simulink model "XSWIFT_cruise"  (R2025b)
settings: Solver=ode4  StartTime=0.0  StopTime=85  FixedStep=0.001  MaxStep=0.001  RelTol=1e-4
InitFcn:
  | [filepath, name] = fileparts(get_param(bdroot, 'FileName'))
  | if strcmp(filepath, pwd) ~= 1
  |     disp(strcat('cambiando el directorio actual a ', filepath))
  |     cd(filepath);
  | end
  | run(strcat(name, '_init'));
  | load("long_cruise.mat");
  | load("lat_cruise.mat")
values from neighbouring files (symbols this model uses):
  d2r = pi/180    (= 0.0174532925199)    [XSWIFT_cruise_init.m]
  data =     [XSWIFT_data.mat]
  init =     [XSWIFT_nav.mat]
  masa = data.mass.zfw + (data.mass.max_takeoff - data.mass.zfw) * mass_frac    [XSWIFT_cruise_init.m]
  nav =     [XSWIFT_nav.mat]
  obs_alpha_la = 20    [implementacion_digital_controles.m]    (also in long_cruise.mat)
  r = rad2deg(x(:,3))    [latero_direccional_LQR.m]
  r2d = 180/pi    (= 57.2957795131)    [XSWIFT_cruise_init.m]
  T_rec = 1/20    (= 0.05)    [XSWIFT_cruise_init.m]
  tau_filtro_lat = 0.3    [lat_cruise.mat]    (also in latero_direccional_LQR.m)
  Tc = 1/25    (= 0.04)    [XSWIFT_cruise_init.m]
  timeSince1970 = 1.3201e+09    (= 1320100000)    [XSWIFT_cruise_init.m]
  x_cg = 0    [XSWIFT_cruise_init.m]
  x_ref = 0    [XSWIFT_cruise_init.m]
undefined symbols (not defined in the file or in its folder): Earth, engine, F, m, MIL, Moderate, s, WGS84, wind
libraries: simulink x6, aerolibconvert2 x4, aerolibasang x4, aerolibfltsims x4, aerolibactuator x3, aerolibwind2 x2, aerolib6dof2 x1, aerolibadyn x1, aerolibatmos2 x1, aerolibanimutils x1, aerolibconvert x1, aerolibobsolete x1
(part 1 of 2)
settings Model: Creator=augusto  LastModifiedBy=Allan
settings SolverCC: AlgebraicLoopSolver=TrustRegion
settings DataIOCC: ReturnWorkspaceOutputs=off
settings DebuggingCC: UnconnectedInputMsg=warning  UnconnectedOutputMsg=warning  UnconnectedLineMsg=warning  ArithmeticOperatorsInVariantConditions=warning
settings ModelReferenceCC: EnableRefExpFcnMdlSchedulingChecks=on
settings SFSimCC: SimUseLocalCustomCode=off  CustomCodeUndefinedFunction=UseInterfaceOnly
settings RTWCC: RTWUseLocalCustomCode=off  GPUComputeCapability=3.5
settings CodeAppCC: StateflowObjectComments=on

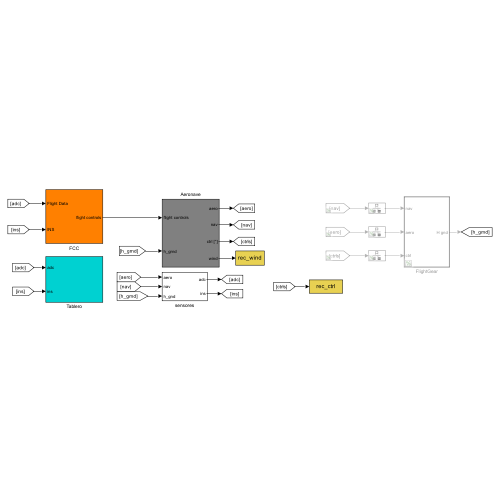
[thumbnail: Simulink's stored preview of the top-level diagram]
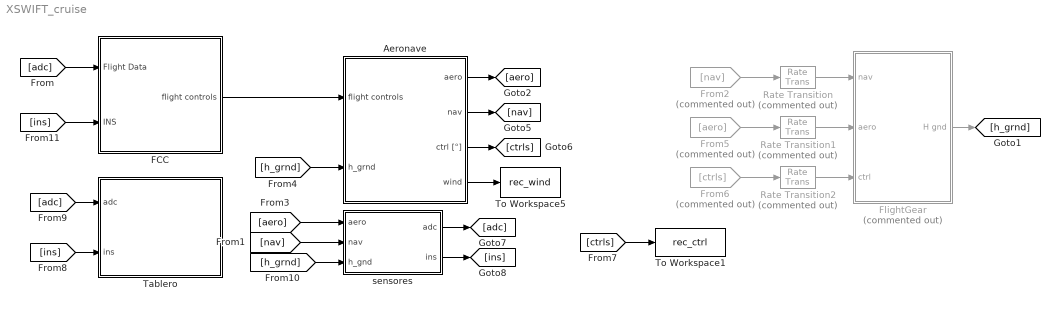
== system XSWIFT_cruise ==
  Aeronave : Subsystem
  FCC : Subsystem
  FlightGear : Subsystem  Commented=on  TreatAsAtomicUnit=on  VariantControl=FlightGearVariant
  From2 : From  Commented=on  GotoTag=nav
  From5 : From  Commented=on  GotoTag=aero
  From6 : From  Commented=on  GotoTag=ctrls
  Rate Transition : RateTransition  Commented=on
  Rate Transition1 : RateTransition  Commented=on
  Rate Transition2 : RateTransition  Commented=on
  Tablero : Subsystem
  To Workspace1 : ToWorkspace  VariableName=rec_ctrl  SampleTime=T_rec
      settings: MaxDataPoints=N_rec
  To Workspace5 : ToWorkspace  VariableName=rec_wind  SampleTime=T_rec
      settings: MaxDataPoints=N_rec
  sensores : Subsystem
  wires:
  FlightGear/1(H gnd) -> [h_grnd]
  From5/1 -> Rate Transition1/1
  Rate Transition2/1 -> FlightGear/3(ctrl)
  Rate Transition1/1 -> FlightGear/2(aero)
  From2/1 -> Rate Transition/1
  From6/1 -> Rate Transition2/1
  Rate Transition/1 -> FlightGear/1(nav)
  [adc] -> FCC/1(Flight Data)
  [ins] -> FCC/2(INS)
  [adc] -> Tablero/1(adc)
  [ins] -> Tablero/2(ins)
  [h_grnd] -> Aeronave/2(h_grnd)
  FCC/1(flight controls) -> Aeronave/1(flight controls)
  Aeronave/3(ctrl [°]) -> [ctrls]
  Aeronave/4(wind) -> To Workspace5/1
  sensores/1(adc) -> [adc]
  sensores/2(ins) -> [ins]
  Aeronave/1(aero) -> [aero]
  Aeronave/2(nav) -> [nav]
  [aero] -> sensores/1(aero)
  [nav] -> sensores/2(nav)
  [h_grnd] -> sensores/3(h_gnd)
  [ctrls] -> To Workspace1/1

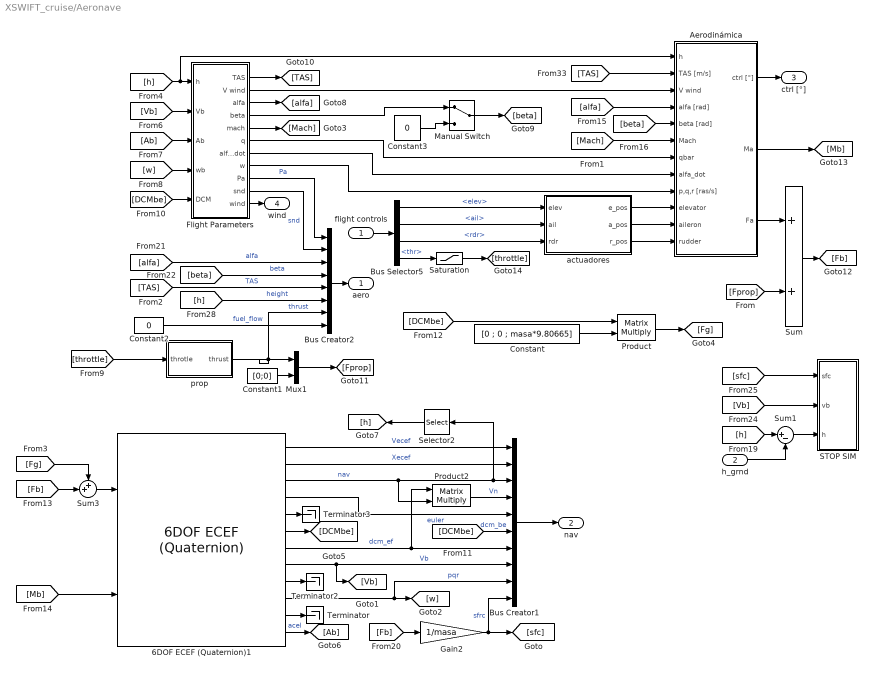
== system XSWIFT_cruise/Aeronave ==
  flight controls : Inport
  h_grnd : Inport  Port=2
  6DOF ECEF (Quaternion)1 : aerolib6dof2/6DOF ECEF (Quaternion)  units=Metric (MKS)  mtype=Fixed  xg_0=init.lla  Vm_0=init.vb  eul_0=init.eul  pm_0=init.wb  mass_0=masa  mass_e=0.5  mass_f=2.0  inertia=inercia  inertia_e=eye(3)  inertia_f=2*eye(3)  vre_flag=on  abi_flag=off  ptype=Earth (WGS84)  R=6378137  F=1/298.257223563  w_E=7292115e-11  angle_in=Internal  LPM0=0  quat_statename=''  pm_statename=''  Vm_statename=''  posfixedframe_statename=''  posinertial_statename=''  LPM_statename=''  mass_statename=''
  Aerodinámica : Subsystem
  Bus Creator1 : BusCreator  Inputs=10
  Bus Creator2 : BusCreator  Inputs=8
  Bus Selector5 : BusSelector  OutputSignals=elev,ail,rdr,thr
  Constant : Constant  Value=[0 ; 0 ; masa*9.80665]
  Constant1 : Constant  Value=[0;0]
  Constant2 : Constant  Value=0
  Constant3 : Constant  Value=0
  Flight Parameters : Subsystem
  Gain2 : Gain  Gain=1/masa
  Manual Switch : ManualSwitch
  Mux1 : Mux  Inputs=2
  Product : Product  Multiplication=Matrix(*)  RndMeth=Zero
  Product2 : Product  Multiplication=Matrix(*)  RndMeth=Zero
  STOP SIM : Subsystem
  Saturation : Saturate  UpperLimit=1  LowerLimit=0
  Selector2 : Selector  InputPortWidth=3  IndexOptions=Index vector (dialog)  Indices=[3]  OutputSizes=1
  Sum : Sum
  Sum1 : Sum  Inputs=|+-
  Sum3 : Sum  Inputs=++|
  Terminator : Terminator
  Terminator2 : Terminator
  Terminator3 : Terminator
  actuadores : Subsystem
  prop : Subsystem
  aero : Outport
  nav : Outport  Port=2
  ctrl [°] : Outport  Port=3
  wind : Outport  Port=4
  wires:
  6DOF ECEF (Quaternion)1/2 -> Bus Creator1/2  "Xecef"
  6DOF ECEF (Quaternion)1/6 -> [DCMbe]
  6DOF ECEF (Quaternion)1/8 -> [Vb], Bus Creator1/8  "Vb"
  6DOF ECEF (Quaternion)1/9 -> Terminator2/1
  6DOF ECEF (Quaternion)1/12 -> [Ab]  "acel"
  Constant/1 -> Product/2
  Constant2/1 -> Bus Creator2/8  "fuel_flow"
  Constant1/1 -> Mux1/2
  [h] -> Aerodinámica/1(h), Flight Parameters/1(h)
  [Vb] -> Flight Parameters/2(Vb)
  Flight Parameters/6(q) -> Aerodinámica/7(qbar)
  Flight Parameters/5(mach) -> [Mach]
  [Mach] -> Aerodinámica/6(Mach)
  Flight Parameters/3(alfa) -> [alfa]
  [alfa] -> Aerodinámica/4(alfa [rad])
  [beta] -> Aerodinámica/5(beta [rad])
  Flight Parameters/2(V wind) -> Aerodinámica/3(V wind)
  Aerodinámica/3(Fa) -> Sum/1
  Flight Parameters/1(TAS) -> [TAS]
  6DOF ECEF (Quaternion)1/4 -> Bus Creator1/5  "euler"
  [Ab] -> Flight Parameters/3(Ab)
  Flight Parameters/7(alfa_dot) -> Aerodinámica/8(alfa_dot)
  Sum/1 -> [Fb]
  6DOF ECEF (Quaternion)1/10 -> Bus Creator1/9, [w]  "pqr"
  [alfa] -> Bus Creator2/3  "alfa"
  [beta] -> Bus Creator2/4  "beta"
  [TAS] -> Bus Creator2/5  "TAS"
  Bus Creator2/1 -> aero/1
  Bus Selector5/4 -> Saturation/1  "<thr>"
  Flight Parameters/8(w) -> Aerodinámica/9(p,q,r [ras/s])
  [w] -> Flight Parameters/4(wb)
  [DCMbe] -> Flight Parameters/5(DCM)
  [DCMbe] -> Bus Creator1/6  "dcm_be"
  Saturation/1 -> [throttle]
  Aerodinámica/2(Ma) -> [Mb]
  6DOF ECEF (Quaternion)1/5 -> Terminator3/1
  6DOF ECEF (Quaternion)1/3 -> Product2/2, Bus Creator1/3, Selector2/1  "nav"
  Aerodinámica/1(ctrl [°]) -> ctrl [°]/1
  Bus Creator1/1 -> nav/1
  Flight Parameters/9(Pa) -> Bus Creator2/1  "Pa"
  6DOF ECEF (Quaternion)1/7 -> Bus Creator1/7, Product2/1  "dcm_ef"
  Product2/1 -> Bus Creator1/4  "Vn"
  6DOF ECEF (Quaternion)1/1 -> Bus Creator1/1  "Vecef"
  flight controls/1 -> Bus Selector5/1
  [h] -> Bus Creator2/6  "height"
  Flight Parameters/10(snd) -> Bus Creator2/2  "snd"
  [Fb] -> Gain2/1
  Gain2/1 -> [sfc], Bus Creator1/10  "sfrc"
  Flight Parameters/11(wind) -> wind/1
  Selector2/1 -> [h]
  [TAS] -> Aerodinámica/2(TAS [m/s])
  Bus Selector5/1 -> actuadores/1(elev)  "<elev>"
  Bus Selector5/2 -> actuadores/2(ail)  "<ail>"
  Bus Selector5/3 -> actuadores/3(rdr)  "<rdr>"
  actuadores/1(e_pos) -> Aerodinámica/10(elevator)
  actuadores/2(a_pos) -> Aerodinámica/11(aileron)
  actuadores/3(r_pos) -> Aerodinámica/12(rudder)
  Product/1 -> [Fg]
  [Fb] -> Sum3/2
  [Fg] -> Sum3/1
  [DCMbe] -> Product/1
  Sum3/1 -> 6DOF ECEF (Quaternion)1/1
  [throttle] -> prop/1(throtle)
  prop/1(thrust) -> Mux1/1, Bus Creator2/7  "thrust"
  [Mb] -> 6DOF ECEF (Quaternion)1/2
  [sfc] -> STOP SIM/1(sfc)
  [Vb] -> STOP SIM/2(vb)
  [Fprop] -> Sum/2
  Mux1/1 -> [Fprop]
  [h] -> Sum1/1
  Sum1/1 -> STOP SIM/3(h)
  h_grnd/1 -> Sum1/2
  6DOF ECEF (Quaternion)1/11 -> Terminator/1
  Manual Switch/1 -> [beta]
  Flight Parameters/4(beta) -> Manual Switch/1
  Constant3/1 -> Manual Switch/2

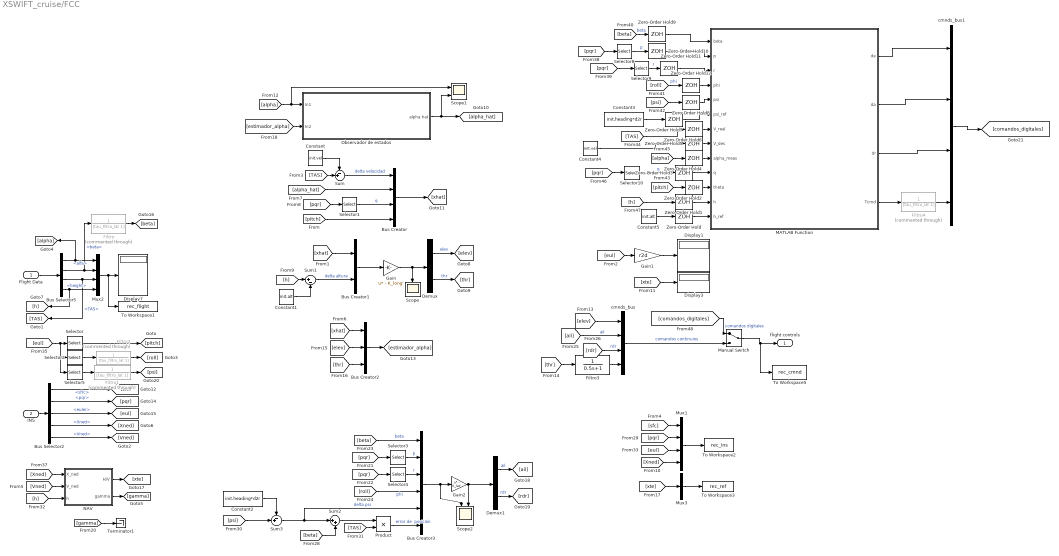
== system XSWIFT_cruise/FCC ==
  Flight Data : Inport
  INS : Inport  Port=2
  Bus Selector2 : BusSelector  OutputSignals=sfrc,pqr,euler,Xned,Vned
  Bus Selector5 : BusSelector  OutputSignals=alfa,beta,TAS,height
  Bus Creator : BusCreator  Inputs=4
  Bus Creator1 : BusCreator  Inputs=2
  Bus Creator2 : BusCreator  Inputs=3
  Bus Creator3 : BusCreator  Inputs=6
  Constant : Constant  Value=init.vel
  Constant1 : Constant  Value=init.alt
  Constant2 : Constant  Value=init.heading*d2r
  Constant3 : Constant  Value=init.heading*d2r
  Constant4 : Constant  Value=init.vel
  Constant5 : Constant  Value=init.alt
  Demux : Demux  Outputs=2
  Demux1 : Demux  Outputs=2
  Display1 : Display
  Display3 : Display
  Display7 : Display
  Filtro{,1..2,4} (4 alike) : TransferFcn  Commented=through  Denominator=[tau_filtro_lat 1]
  Filtro3 : TransferFcn  Denominator=[0.5 1]
  Gain : Gain  Gain=- K_long'  Multiplication=Matrix(u*K)
  Gain1 : Gain  Gain=r2d
  Gain2 : Gain  Gain=- K_lat'  Multiplication=Matrix(u*K)
  MATLAB Function : MATLAB Function  TreatAsAtomicUnit=on
  Manual Switch : ManualSwitch
  Mux1 : Mux
  Mux2 : Mux
  Mux3 : Mux  Inputs=1
  NAV : Subsystem
  Observador de estados : Subsystem
  Product : Product
  Scope : Scope
      settings: ActiveDisplayYMinimum=-0.63580956795157817  ActiveDisplayYMaximum=2.7800022979084402
  Scope1 : Scope  NumInputPorts=2
      settings: ActiveDisplayYMinimum=-0.053966559568766573  ActiveDisplayYMaximum=-0.02656502251691319  DataLoggingVariableName=ScopeData2
  Scope2 : Scope  NumInputPorts=2
      settings: ActiveDisplayYMinimum=-6.3589608284384154  ActiveDisplayYMaximum=1.5540132529438384  DataLoggingVariableName=ScopeData3
  Selector : Selector  InputPortWidth=3  IndexOptions=Index vector (dialog)  Indices=2  OutputSizes=1
  Selector1 : Selector  InputPortWidth=3  IndexOptions=Index vector (dialog)  Indices=2  OutputSizes=1
  Selector10 : Selector  InputPortWidth=3  IndexOptions=Index vector (dialog)  Indices=2  OutputSizes=1
  Selector2 : Selector  InputPortWidth=3  IndexOptions=Index vector (dialog)  Indices=1  OutputSizes=1
  Selector3 : Selector  InputPortWidth=3  IndexOptions=Index vector (dialog)  Indices=1  OutputSizes=1
  Selector4 : Selector  InputPortWidth=3  IndexOptions=Index vector (dialog)  Indices=3  OutputSizes=1
  Selector5 : Selector  InputPortWidth=3  IndexOptions=Index vector (dialog)  Indices=3  OutputSizes=1
  Selector8 : Selector  InputPortWidth=3  IndexOptions=Index vector (dialog)  Indices=1  OutputSizes=1
  Selector9 : Selector  InputPortWidth=3  IndexOptions=Index vector (dialog)  Indices=3  OutputSizes=1
  Sum : Sum  Inputs=-+|
  Sum1 : Sum  Inputs=|+-
  Sum2 : Sum  Inputs=|++
  Sum3 : Sum  Inputs=-+|
  Terminator1 : Terminator
  To Workspace1 : ToWorkspace  VariableName=rec_flight  SampleTime=T_rec
      settings: MaxDataPoints=N_rec
  To Workspace2 : ToWorkspace  VariableName=rec_ins  SampleTime=T_rec
      settings: MaxDataPoints=N_rec
  To Workspace3 : ToWorkspace  VariableName=rec_ref  SampleTime=T_rec
      settings: MaxDataPoints=N_rec
  To Workspace5 : ToWorkspace  VariableName=rec_cmnd  SampleTime=T_rec
      settings: MaxDataPoints=N_rec
  Zero-Order Hold{,1..12} (13 alike) : ZeroOrderHold  SampleTime=-1
  cmnds_bus : BusCreator  Inputs=4  OutDataTypeStr=Bus: cmnds_bus
      settings: InheritFromInputs=off
  cmnds_bus1 : BusCreator  Inputs=4  OutDataTypeStr=Bus: cmnds_bus
      settings: InheritFromInputs=off
  flight controls : Outport
  wires:
  Mux2/1 -> To Workspace1/1, Display7/1
  Bus Selector5/2 -> Filtro/1, Mux2/2  "<beta>"
  Bus Selector5/1 -> [alpha], Mux2/1  "<alfa>"
  Bus Selector5/3 -> [TAS], Mux2/3  "<TAS>"
  Bus Selector5/4 -> [h], Mux2/4  "<height>"
  INS/1 -> Bus Selector2/1
  Flight Data/1 -> Bus Selector5/1
  [rdr] -> cmnds_bus/3  "rdr"
  [ail] -> cmnds_bus/2  "ail"
  Bus Selector2/3 -> [eul]  "<euler>"
  Selector/1 -> [pitch]
  Bus Selector2/1 -> [sfc]  "<sfrc>"
  Bus Selector2/2 -> [pqr]  "<pqr>"
  [Xned] -> Mux1/4
  [xte] -> Display3/1
  Mux3/1 -> To Workspace3/1
  [xte] -> Mux3/1
  Bus Selector2/4 -> [Xned]  "<Xned>"
  Mux1/1 -> To Workspace2/1
  [sfc] -> Mux1/1
  [pqr] -> Mux1/2
  [eul] -> Mux1/3
  Gain1/1 -> Display1/1
  [eul] -> Gain1/1
  [pitch] -> Bus Creator/4
  [Xned] -> NAV/1(X_ned)
  NAV/1(H/V) -> [xte]
  [h] -> NAV/3(h)
  Bus Selector2/5 -> [Vned]  "<Vned>"
  [Vned] -> NAV/2(V_ned)
  NAV/2(gamma) -> [gamma]
  [alpha_hat] -> Bus Creator/2
  [pqr] -> Selector1/1
  Selector1/1 -> Bus Creator/3  "q"
  Bus Creator1/1 -> Gain/1
  [h] -> Sum1/1
  Gain/1 -> Scope/1, Demux/1
  Demux/1 -> [elev]  "elev"
  Demux/2 -> [thr]  "thr"
  [TAS] -> Sum/2
  Sum/1 -> Bus Creator/1  "delta velocidad"
  Sum1/1 -> Bus Creator1/2  "delta altura"
  Constant1/1 -> Sum1/2
  [elev] -> cmnds_bus/1
  [thr] -> Filtro3/1
  Bus Creator/1 -> [xhat]
  [xhat] -> Bus Creator1/1
  [xhat] -> Bus Creator2/1
  [elev] -> Bus Creator2/2
  [thr] -> Bus Creator2/3
  Bus Creator2/1 -> [estimador_alpha]
  [alpha] -> Scope1/1, Observador de estados/1(In1)
  Observador de estados/1(alpha hat) -> [alpha_hat], Scope1/2
  [estimador_alpha] -> Observador de estados/2(In2)
  [gamma] -> Terminator1/1
  Constant/1 -> Sum/1
  [pqr] -> Selector3/1
  [pqr] -> Selector4/1
  [beta] -> Bus Creator3/1  "beta"
  Selector3/1 -> Bus Creator3/2  "p"
  Selector4/1 -> Bus Creator3/3  "r"
  [roll] -> Bus Creator3/4  "phi"
  Demux1/2 -> [rdr]  "rdr"
  Gain2/1 -> Demux1/1, Scope2/2
  Demux1/1 -> [ail]  "ail"
  Bus Creator3/1 -> Scope2/1, Gain2/1
  [eul] -> Selector5/1, Selector2/1, Selector/1
  [beta] -> Sum2/2
  Sum2/1 -> Product/1
  [TAS] -> Product/2
  [psi] -> Sum3/2
  Constant2/1 -> Sum3/1
  Sum3/1 -> Sum2/1, Bus Creator3/5  "delta psi"
  Product/1 -> Bus Creator3/6  "error de  posición"
  Filtro/1 -> [beta]
  Selector5/1 -> Filtro1/1
  Filtro1/1 -> [psi]
  Selector2/1 -> Filtro2/1
  Filtro2/1 -> [roll]
  [pqr] -> Selector8/1
  [roll] -> Zero-Order Hold12/1  "phi"
  Selector9/1 -> Zero-Order Hold11/1  "r"
  [beta] -> Zero-Order Hold9/1  "beta"
  Selector8/1 -> Zero-Order Hold10/1  "p"
  [pqr] -> Selector9/1
  [psi] -> Zero-Order Hold8/1
  Constant3/1 -> Zero-Order Hold7/1
  Constant4/1 -> Zero-Order Hold5/1
  [pqr] -> Selector10/1
  [TAS] -> Zero-Order Hold6/1
  [pitch] -> Zero-Order Hold2/1
  Selector10/1 -> Zero-Order Hold3/1  "q"
  [alpha] -> Zero-Order Hold4/1
  [h] -> Zero-Order Hold1/1
  Constant5/1 -> Zero-Order Hold/1
  MATLAB Function/4(Tcmd) -> Filtro4/1
  cmnds_bus1/1 -> [comandos_digitales]
  [comandos_digitales] -> Manual Switch/1  "comandos digitales"
  Zero-Order Hold/1 -> MATLAB Function/13(h_ref)
  Zero-Order Hold1/1 -> MATLAB Function/12(h)
  Zero-Order Hold2/1 -> MATLAB Function/11(theta)
  Zero-Order Hold3/1 -> MATLAB Function/10(q)
  Zero-Order Hold4/1 -> MATLAB Function/9(alpha_meas)
  Zero-Order Hold5/1 -> MATLAB Function/8(V_des)
  Zero-Order Hold6/1 -> MATLAB Function/7(V_real)
  Zero-Order Hold7/1 -> MATLAB Function/6(psi_ref)
  Zero-Order Hold8/1 -> MATLAB Function/5(psi)
  Zero-Order Hold9/1 -> MATLAB Function/1(beta)
  Zero-Order Hold10/1 -> MATLAB Function/2(p)
  Zero-Order Hold11/1 -> MATLAB Function/3(r)
  Zero-Order Hold12/1 -> MATLAB Function/4(phi)
  MATLAB Function/1(de) -> cmnds_bus1/1
  MATLAB Function/2(da) -> cmnds_bus1/2
  MATLAB Function/3(dr) -> cmnds_bus1/3
  cmnds_bus/1 -> Manual Switch/2  "comandos continuios"
  Manual Switch/1 -> To Workspace5/1, flight controls/1
  Filtro3/1 -> cmnds_bus/4
  Filtro4/1 -> cmnds_bus1/4

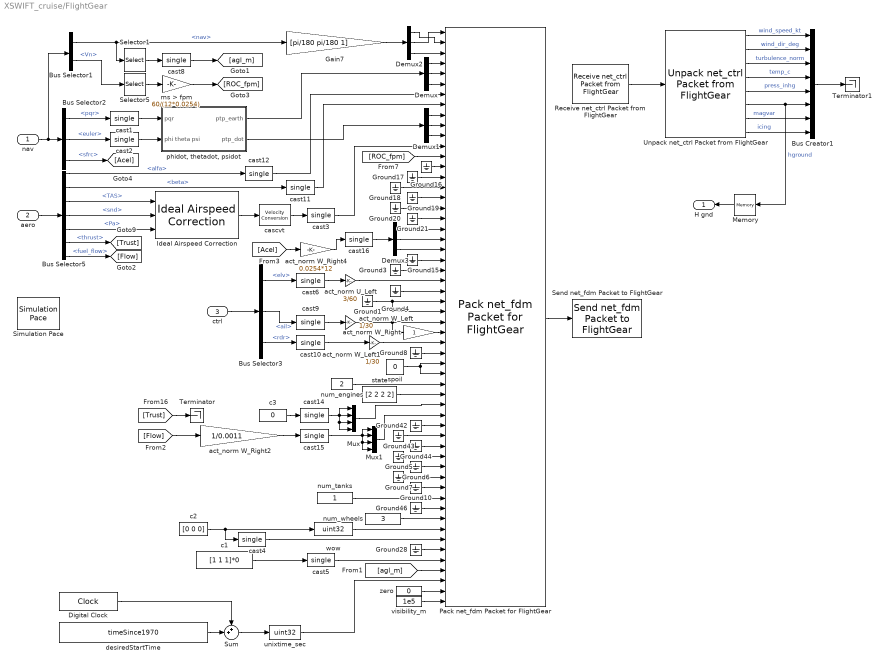
== system XSWIFT_cruise/FlightGear ==
  nav : Inport  SampleTime=Tc
  aero : Inport  Port=2  SampleTime=Tc
  ctrl : Inport  Port=3  SampleTime=Tc
  Bus Creator1 : BusCreator  Inputs=8
  Bus Selector1 : BusSelector  OutputSignals=nav,Vn
  Bus Selector2 : BusSelector  OutputSignals=pqr,euler,sfrc
  Bus Selector3 : BusSelector  OutputSignals=elv,ail,rdr
  Bus Selector5 : BusSelector  OutputSignals=alfa,beta,TAS,snd,Pa,thrust,fuel_flow
  Demux{,1..3} (4 alike) : Demux  Outputs=3
  Digital Clock : DigitalClock  SampleTime=Tc
  Gain7 : Gain  Gain=[pi/180 pi/180 1]
  Ground{1,3..8,10,15..21,28,42..44,46} (20 alike) : Ground
  Ideal Airspeed Correction : aerolibasang/Ideal Airspeed Correction  units=Metric (MKS)  vel_in=TAS  vel_out_tas=CAS  vel_out_eas=CAS  vel_out_cas=TAS  method=Table Lookup  SubOnly=off  action=Warning
  Memory : Memory  InheritSampleTime=on
  Mux : Mux
  Mux1 : Mux
  Pack net_fdm Packet for FlightGear : aerolibfltsims/Pack net_fdm Packet for FlightGear  FlightGearVersion=v2016.3  ShowPositionAttitudeInputs=on  ShowVelocityAccelerationInputs=on  ShowControlSurfacePositionInputs=on  ShowEngineFuelInputs=on  ShowLandingGearInputs=on  ShowEnvironmentInputs=on  SampleTime=Tc  packetVersion=24
  Receive net_ctrl Packet from FlightGear : aerolibfltsims/Receive net_ctrl Packet from FlightGear  FlightGearVersion=v3.0  ReceiveAddress=127.0.0.1  ReceivePort=5505  ReceiveWidth=744  varLen=off  SampleTime=Tc  packetFlag=off
      settings: AttributesFormatString=Version Selected:\n%<FlightGearVersion>
  Selector1 : Selector  InputPortWidth=3  IndexOptions=Index vector (dialog)  Indices=3  OutputSizes=1
  Selector5 : Selector  InputPortWidth=3  IndexOptions=Index vector (dialog)  Indices=3  OutputSizes=1
  Send net_fdm Packet to FlightGear : aerolibfltsims/Send net_fdm Packet to FlightGear  DestinationIpAddress=127.0.0.1  DestinationPort=5502  LocalIpPort=-1  varLen=off  SampleTime=Tc
  Simulation Pace : aerolibanimutils/Simulation Pace  SimulationPace=1  SleepMode=MATLAB Thread  OutputPaceError=off  SampleTime=Tc
      settings: AttributesFormatString=%<SimulationPace> sec/sec
  Sum : Sum  Inputs=++|
  Terminator : Terminator
  Terminator1 : Terminator
  Unpack net_ctrl Packet from FlightGear : aerolibfltsims/Unpack net_ctrl Packet from FlightGear  FlightGearVersion=v2016.3  ShowControlSurfacePositionOutputs=off  ShowEngineFuelOutputs=off  ShowLandingGearOutputs=off  ShowAvionicOutputs=off  ShowEnvironmentOutputs=on  SampleTime=Tc  packetVersion=27
      settings: AttributesFormatString=Version Selected: %<FlightGearVersion>
  act_norm U_Left : Gain  Gain=3/60
      settings: AttributesFormatString=%<Gain>
  act_norm W_Left : Gain  Gain=1/30
      settings: AttributesFormatString=%<Gain>
  act_norm W_Left1 : Gain  Gain=1/30
      settings: AttributesFormatString=%<Gain>
  act_norm W_Right : Gain
      settings: AttributesFormatString=%<Gain>
  act_norm W_Right2 : Gain  Gain=1/0.0011
      settings: AttributesFormatString=%<Gain>
  act_norm W_Right4 : Gain  Gain=0.0254*12
      settings: AttributesFormatString=%<Gain>
  c1 : Constant  Value=[1 1 1]*0  OutDataTypeStr=uint32
  c2 : Constant  Value=[0 0 0]  OutDataTypeStr=uint32
  c3 : Constant  Value=0  OutDataTypeStr=uint32
  cascvt : aerolibconvert/Velocity Conversion  IU=m/s  OU=kts
  cast{1..6,8..12,14..16} (14 alike) : DataTypeConversion  OutDataTypeStr=single  RndMeth=Floor
  desiredStartTime : Constant  Value=timeSince1970
  ms > fpm : Gain  Gain=60/(12*0.0254)  OutDataTypeStr=single
  num_engines : Constant  Value=2  OutDataTypeStr=uint32
  num_tanks : Constant  OutDataTypeStr=uint32
  num_wheels : Constant  Value=3  OutDataTypeStr=uint32
  "phidot, thetadot, psidot" : Subsystem
  spoil : Constant  Value=0  OutDataTypeStr=single
  state : Constant  Value=[2 2 2 2]  OutDataTypeStr=uint32
  unixtime_sec : DataTypeConversion  OutDataTypeStr=uint32  RndMeth=Floor
  visibility_m : Constant  Value=1e5  OutDataTypeStr=single
  wow : DataTypeConversion  OutDataTypeStr=uint32  RndMeth=Floor
  zero : Constant  Value=0  OutDataTypeStr=int32
  H gnd : Outport
  wires:
  Unpack net_ctrl Packet from FlightGear/6 -> Memory/1, Bus Creator1/6  "hground"
  Unpack net_ctrl Packet from FlightGear/8 -> Bus Creator1/8  "icing"
  Unpack net_ctrl Packet from FlightGear/7 -> Bus Creator1/7  "magvar"
  Unpack net_ctrl Packet from FlightGear/5 -> Bus Creator1/5  "press_inhg"
  Unpack net_ctrl Packet from FlightGear/4 -> Bus Creator1/4  "temp_c"
  Unpack net_ctrl Packet from FlightGear/3 -> Bus Creator1/3  "turbulence_norm"
  Unpack net_ctrl Packet from FlightGear/2 -> Bus Creator1/2  "wind_dir_deg"
  Unpack net_ctrl Packet from FlightGear/1 -> Bus Creator1/1  "wind_speed_kt"
  Receive net_ctrl Packet from FlightGear/1 -> Unpack net_ctrl Packet from FlightGear/1
  Ground1/1 -> Pack net_fdm Packet for FlightGear/28, Pack net_fdm Packet for FlightGear/27
  Ground10/1 -> Pack net_fdm Packet for FlightGear/45
  wow/1 -> Pack net_fdm Packet for FlightGear/49
  cast9/1 -> act_norm W_Left/1
  Ground8/1 -> Pack net_fdm Packet for FlightGear/32
  act_norm W_Right/1 -> Pack net_fdm Packet for FlightGear/30
  act_norm W_Left/1 -> act_norm W_Right/1, Pack net_fdm Packet for FlightGear/29
  Ground4/1 -> Pack net_fdm Packet for FlightGear/26
  Ground7/1 -> Pack net_fdm Packet for FlightGear/44
  Ground6/1 -> Pack net_fdm Packet for FlightGear/43
  Ground5/1 -> Pack net_fdm Packet for FlightGear/42
  Ground3/1 -> Pack net_fdm Packet for FlightGear/24
  Demux1/3 -> Pack net_fdm Packet for FlightGear/11
  Demux1/2 -> Pack net_fdm Packet for FlightGear/10
  Demux1/1 -> Pack net_fdm Packet for FlightGear/9
  act_norm U_Left/1 -> Pack net_fdm Packet for FlightGear/25
  [agl_m] -> Pack net_fdm Packet for FlightGear/53
  Demux/3 -> Pack net_fdm Packet for FlightGear/6
  Demux/2 -> Pack net_fdm Packet for FlightGear/5
  Demux/1 -> Pack net_fdm Packet for FlightGear/4
  cast4/1 -> Pack net_fdm Packet for FlightGear/50
  cast6/1 -> act_norm U_Left/1
  cast5/1 -> Pack net_fdm Packet for FlightGear/52
  ms > fpm/1 -> [ROC_fpm]
  [ROC_fpm] -> Pack net_fdm Packet for FlightGear/13
  Bus Selector5/5 -> Ideal Airspeed Correction/3  "<Pa>"
  Bus Selector5/4 -> Ideal Airspeed Correction/2  "<snd>"
  Bus Selector2/2 -> cast2/1  "<euler>"
  Bus Selector2/1 -> cast1/1  "<pqr>"
  "phidot, thetadot, psidot"/2(ptp_dot) -> Demux1/1
  "phidot, thetadot, psidot"/1(ptp_earth) -> Demux/1
  cast3/1 -> Pack net_fdm Packet for FlightGear/12
  cast1/1 -> "phidot, thetadot, psidot"/1(pqr)
  cast2/1 -> "phidot, thetadot, psidot"/2(phi theta psi)
  visibility_m/1 -> Pack net_fdm Packet for FlightGear/56
  zero/1 -> Pack net_fdm Packet for FlightGear/55
  unixtime_sec/1 -> Pack net_fdm Packet for FlightGear/54
  Sum/1 -> unixtime_sec/1
  desiredStartTime/1 -> Sum/2
  Digital Clock/1 -> Sum/1
  cascvt/1 -> cast3/1
  Ideal Airspeed Correction/1 -> cascvt/1
  Ground28/1 -> Pack net_fdm Packet for FlightGear/51
  num_wheels/1 -> Pack net_fdm Packet for FlightGear/48
  Ground46/1 -> Pack net_fdm Packet for FlightGear/47
  num_tanks/1 -> Pack net_fdm Packet for FlightGear/46
  Ground44/1 -> Pack net_fdm Packet for FlightGear/41
  Ground43/1 -> Pack net_fdm Packet for FlightGear/40
  Ground42/1 -> Pack net_fdm Packet for FlightGear/39
  state/1 -> Pack net_fdm Packet for FlightGear/36
  num_engines/1 -> Pack net_fdm Packet for FlightGear/35
  Ground15/1 -> Pack net_fdm Packet for FlightGear/23
  Demux3/3 -> Pack net_fdm Packet for FlightGear/22
  Demux3/2 -> Pack net_fdm Packet for FlightGear/21
  Demux3/1 -> Pack net_fdm Packet for FlightGear/20
  Ground21/1 -> Pack net_fdm Packet for FlightGear/19
  Ground20/1 -> Pack net_fdm Packet for FlightGear/18
  Ground19/1 -> Pack net_fdm Packet for FlightGear/17
  Ground18/1 -> Pack net_fdm Packet for FlightGear/16
  Ground17/1 -> Pack net_fdm Packet for FlightGear/15
  Ground16/1 -> Pack net_fdm Packet for FlightGear/14
  Bus Selector3/1 -> cast6/1  "<elv>"
  Bus Selector3/2 -> cast9/1  "<ail>"
  cast10/1 -> act_norm W_Left1/1
  Bus Selector3/3 -> cast10/1  "<rdr>"
  act_norm W_Left1/1 -> Pack net_fdm Packet for FlightGear/31
  Demux2/3 -> Pack net_fdm Packet for FlightGear/3
  Bus Selector1/1 -> Gain7/1, Selector1/1  "<nav>"
  Bus Selector5/3 -> Ideal Airspeed Correction/1  "<TAS>"
  Selector5/1 -> ms > fpm/1
  Bus Selector1/2 -> Selector5/1  "<Vn>"
  c2/1 -> cast4/1, wow/1
  Selector1/1 -> cast8/1
  cast8/1 -> [agl_m]
  Gain7/1 -> Demux2/1
  Pack net_fdm Packet for FlightGear/1 -> Send net_fdm Packet to FlightGear/1
  Demux2/2 -> Pack net_fdm Packet for FlightGear/1
  Demux2/1 -> Pack net_fdm Packet for FlightGear/2
  Bus Selector5/2 -> cast11/1  "<beta>"
  cast12/1 -> Pack net_fdm Packet for FlightGear/7
  cast11/1 -> Pack net_fdm Packet for FlightGear/8
  Bus Selector5/1 -> cast12/1  "<alfa>"
  spoil/1 -> Pack net_fdm Packet for FlightGear/34, Pack net_fdm Packet for FlightGear/33
  Memory/1 -> H gnd/1
  Bus Creator1/1 -> Terminator1/1
  nav/1 -> Bus Selector2/1, Bus Selector1/1
  aero/1 -> Bus Selector5/1
  ctrl/1 -> Bus Selector3/1
  Bus Selector5/6 -> [Trust]  "<thrust>"
  Bus Selector5/7 -> [Flow]  "<fuel_flow>"
  act_norm W_Right2/1 -> cast15/1
  [Flow] -> act_norm W_Right2/1
  Bus Selector2/3 -> [Acel]  "<sfrc>"
  cast16/1 -> Demux3/1
  [Acel] -> act_norm W_Right4/1
  act_norm W_Right4/1 -> cast16/1
  cast14/1 -> Mux/4, Mux/3, Mux/2, Mux/1
  Mux/1 -> Pack net_fdm Packet for FlightGear/37
  cast15/1 -> Mux1/4, Mux1/3, Mux1/1, Mux1/2
  Mux1/1 -> Pack net_fdm Packet for FlightGear/38
  c3/1 -> cast14/1
  [Trust] -> Terminator/1
  c1/1 -> cast5/1

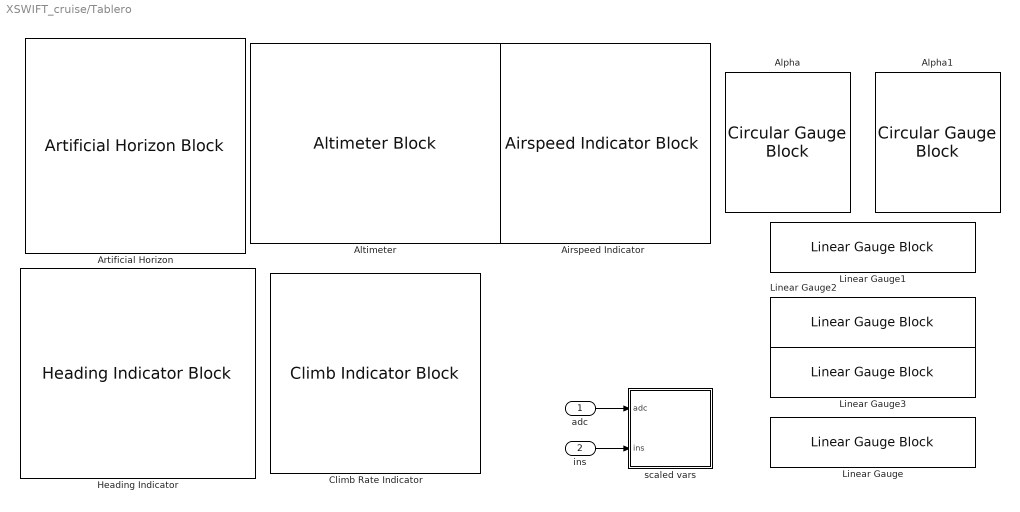
== system XSWIFT_cruise/Tablero ==
  adc : Inport
  ins : Inport  Port=2
  Airspeed Indicator : AirspeedIndicatorBlock  ScaleMin=0  ScaleMax=90
  Alpha : CircularGaugeBlock  ScaleMin=-10  ScaleMax=20  FontColor=[0.0, 0.0, 0.0]
  Alpha1 : CircularGaugeBlock  ScaleMin=-5  ScaleMax=5  FontColor=[0.0, 0.0, 0.0]
  Altimeter : AltimeterBlock
  Artificial Horizon : ArtificialHorizonBlock
  Climb Rate Indicator : ClimbIndicatorBlock  ScaleMax=1000
  Heading Indicator : HeadingIndicatorBlock
  Linear Gauge : LinearGaugeBlock  ScaleMax=1  TickInterval=0.2  FontColor=[0.0, 0.0, 0.0]
  Linear Gauge1 : LinearGaugeBlock  ScaleMin=-1  ScaleMax=1  TickInterval=0.5  FontColor=[0.0, 0.0, 0.0]
  Linear Gauge2 : LinearGaugeBlock  ScaleMin=-1  ScaleMax=1  TickInterval=0.5  FontColor=[0.0, 0.0, 0.0]
  Linear Gauge3 : LinearGaugeBlock  ScaleMin=-1  ScaleMax=1  TickInterval=0.5  FontColor=[0.0, 0.0, 0.0]
  scaled vars : Subsystem
  wires:
  adc/1 -> scaled vars/1(adc)
  ins/1 -> scaled vars/2(ins)

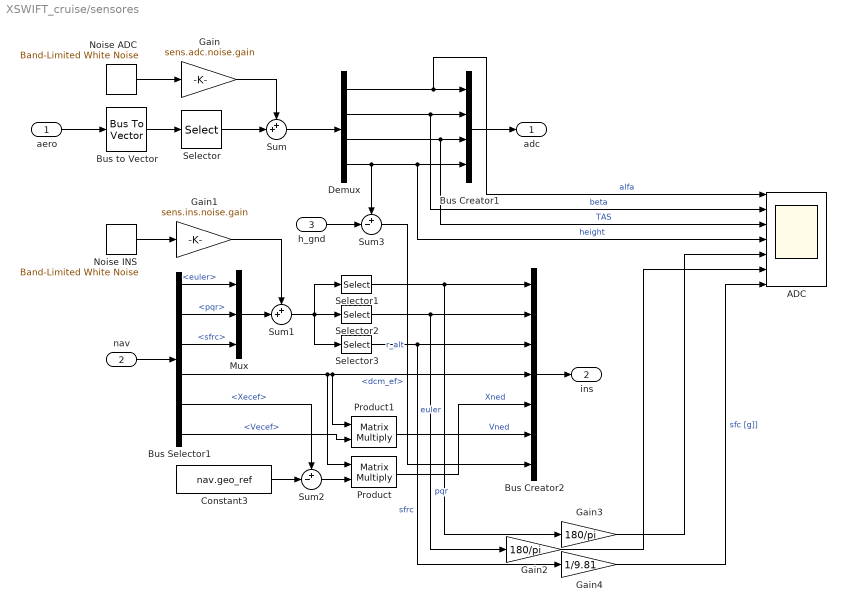
== system XSWIFT_cruise/sensores ==
  aero : Inport
  nav : Inport  Port=2
  h_gnd : Inport  Port=3
  ADC : Scope  NumInputPorts=7
      settings: ActiveDisplayYMinimum=-0.096081502545540057  ActiveDisplayYMaximum=0.11900905583839336
  Bus Creator1 : BusCreator  Inputs=4
  Bus Creator2 : BusCreator  Inputs=7  OutDataTypeStr=Bus: ins_bus
      settings: InheritFromInputs=off
  Bus Selector1 : BusSelector  OutputSignals=euler,pqr,sfrc,dcm_ef,Xecef,Vecef
  Bus to Vector : BusToVector
  Constant3 : Constant  Value=nav.geo_ref
  Demux : Demux
  Gain : Gain  Gain=sens.adc.noise.gain
  Gain1 : Gain  Gain=sens.ins.noise.gain
  Gain2 : Gain  Gain=180/pi
  Gain3 : Gain  Gain=180/pi
  Gain4 : Gain  Gain=1/9.81
  Mux : Mux  Inputs=3
  Noise ADC : simulink/Sources/Band-Limited White Noise  Cov=[0.01]  Ts=0.01  seed=sens.adc.noise.seeds
  Noise INS : simulink/Sources/Band-Limited White Noise  Cov=[0.01]  Ts=0.01  seed=sens.ins.noise.seeds
  Product : Product  Multiplication=Matrix(*)  RndMeth=Zero
  Product1 : Product  Multiplication=Matrix(*)  RndMeth=Zero
  Selector : Selector  InputPortWidth=8  IndexOptions=Index vector (dialog)  Indices=[3 4 5 6]  OutputSizes=1
  Selector1 : Selector  InputPortWidth=9  IndexOptions=Index vector (dialog)  Indices=1:3  OutputSizes=1
  Selector2 : Selector  InputPortWidth=9  IndexOptions=Index vector (dialog)  Indices=4:6  OutputSizes=1
  Selector3 : Selector  InputPortWidth=9  IndexOptions=Index vector (dialog)  Indices=7:9  OutputSizes=1
  Sum : Sum  Inputs=++|
  Sum1 : Sum  Inputs=++|
  Sum2 : Sum  Inputs=+-|
  Sum3 : Sum  Inputs=+-|
  adc : Outport
  ins : Outport  Port=2
  wires:
  nav/1 -> Bus Selector1/1
  Bus Creator1/1 -> adc/1
  aero/1 -> Bus to Vector/1
  Noise ADC/1 -> Gain/1
  Bus to Vector/1 -> Selector/1
  Gain/1 -> Sum/1
  Demux/1 -> ADC/1, Bus Creator1/1  "alfa"
  Demux/2 -> ADC/2, Bus Creator1/2  "beta"
  Demux/3 -> ADC/3, Bus Creator1/3  "TAS"
  Sum/1 -> Demux/1
  Demux/4 -> Sum3/1, ADC/4, Bus Creator1/4  "height"
  Selector/1 -> Sum/2
  Bus Creator2/1 -> ins/1
  Selector1/1 -> Gain3/1, Bus Creator2/1  "euler"
  Selector2/1 -> Gain2/1, Bus Creator2/2  "pqr"
  Selector3/1 -> Gain4/1, Bus Creator2/3  "sfrc"
  Bus Selector1/1 -> Mux/1  "<euler>"
  Bus Selector1/2 -> Mux/2  "<pqr>"
  Bus Selector1/3 -> Mux/3  "<sfrc>"
  Gain1/1 -> Sum1/1
  Mux/1 -> Sum1/2
  Noise INS/1 -> Gain1/1
  Sum1/1 -> Selector3/1, Selector2/1, Selector1/1
  Gain3/1 -> ADC/5
  Gain2/1 -> ADC/6
  Gain4/1 -> ADC/7  "sfc [g]]"
  Bus Selector1/5 -> Sum2/1  "<Xecef>"
  Bus Selector1/4 -> Product/1, Product1/1, Bus Creator2/4  "<dcm_ef>"
  Constant3/1 -> Sum2/2
  Sum2/1 -> Product/2
  Product/1 -> Bus Creator2/5  "Xned"
  Bus Selector1/6 -> Product1/2  "<Vecef>"
  Product1/1 -> Bus Creator2/6  "Vned"
  h_gnd/1 -> Sum3/2
  Sum3/1 -> Bus Creator2/7  "r_alt"

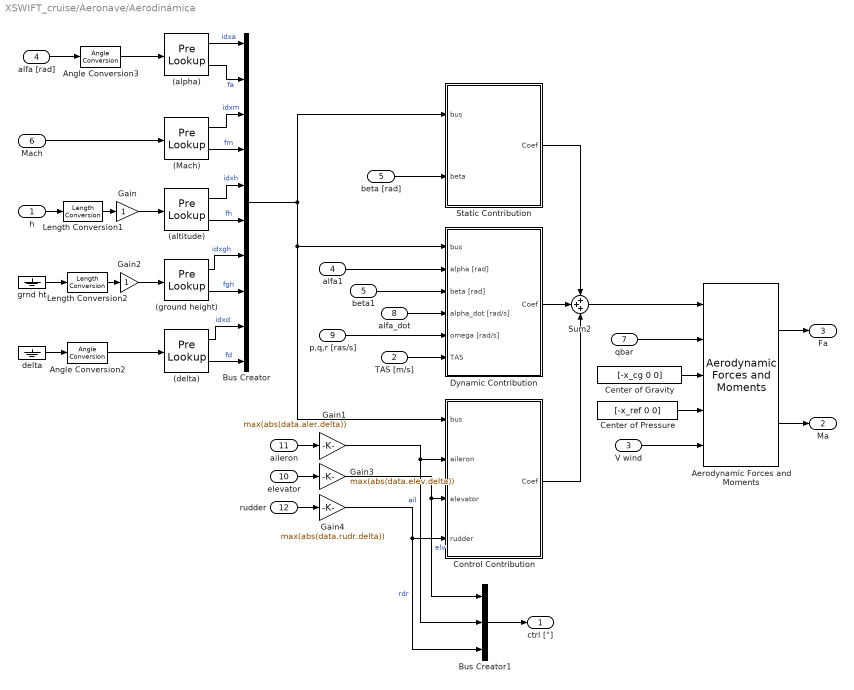
== system XSWIFT_cruise/Aeronave/Aerodinámica ==
  h : Inport
  TAS [m/s] : Inport  Port=2
  V wind : Inport  Port=3
  alfa [rad] : Inport  Port=4
  beta [rad] : Inport  Port=5
  Mach : Inport  Port=6
  qbar : Inport  Port=7
  alfa_dot : Inport  Port=8
  p,q,r [ras/s] : Inport  Port=9
  elevator : Inport  Port=10
  aileron : Inport  Port=11
  rudder : Inport  Port=12
  (Mach) : PreLookup  BreakpointsData=0:2  BeginIndexSearchUsingPreviousIndexResult=on  ExtrapMethod=Linear  IndexDataTypeStr=int32  FractionDataTypeStr=double
  (alpha) : PreLookup  BreakpointsData=data.alpha  BeginIndexSearchUsingPreviousIndexResult=on  ExtrapMethod=Linear  IndexDataTypeStr=int32  FractionDataTypeStr=double
  (altitude) : PreLookup  BreakpointsData=0:2  BeginIndexSearchUsingPreviousIndexResult=on  ExtrapMethod=Linear  IndexDataTypeStr=int32  FractionDataTypeStr=double
  (delta) : PreLookup  BreakpointsData=[0:2]  BeginIndexSearchUsingPreviousIndexResult=on  ExtrapMethod=Linear  IndexDataTypeStr=int32  FractionDataTypeStr=double
  (ground height) : PreLookup  BreakpointsData=[0:2]  BeginIndexSearchUsingPreviousIndexResult=on  ExtrapMethod=Linear  IndexDataTypeStr=int32  FractionDataTypeStr=double
  Aerodynamic Forces and Moments : aerolibadyn/Aerodynamic Forces and Moments   inputAxes=Stability  outputForceAxes=Body  outputMomentAxes=Body  S=data.sref  b=data.blref  cbar=data.cbar
  Angle Conversion2 : aerolibconvert2/Angle Conversion  IU=rad  OU=deg
  Angle Conversion3 : aerolibconvert2/Angle Conversion  IU=rad  OU=deg
  Bus Creator : BusCreator  Inputs=10
  Bus Creator1 : BusCreator  Inputs=3
  Center of Gravity : Constant  Value=[-x_cg 0 0]  SampleTime=0
  Center of Pressure : Constant  Value=[-x_ref 0 0]  SampleTime=0
  Control Contribution : Subsystem  mask(Static Contribution 1-D){}
  Dynamic Contribution : Subsystem  mask(Dynamic Contribution 1-D){}
  Gain : Gain
  Gain1 : Gain  Gain=max(abs(data.aler.delta))
  Gain2 : Gain
  Gain3 : Gain  Gain=max(abs(data.elev.delta))
  Gain4 : Gain  Gain=max(abs(data.rudr.delta))
  Length Conversion1 : aerolibconvert2/Length Conversion  IU=m  OU=m
  Length Conversion2 : aerolibconvert2/Length Conversion  IU=m  OU=m
  Static Contribution : Subsystem  mask(Static Contribution 1-D){}
  Sum2 : Sum  Inputs=+++
  alfa1 : InportShadow  Port=4
  beta1 : InportShadow  Port=5
  delta : Ground
  grnd ht : Ground
  ctrl [°] : Outport
  Ma : Outport  Port=2
  Fa : Outport  Port=3
  wires:
  beta [rad]/1 -> Static Contribution/2(beta)
  (alpha)/2 -> Bus Creator/2  "fa"
  (Mach)/2 -> Bus Creator/4  "fm"
  (altitude)/2 -> Bus Creator/6  "fh"
  (altitude)/1 -> Bus Creator/5  "idxh"
  (ground height)/2 -> Bus Creator/8  "fgh"
  (ground height)/1 -> Bus Creator/7  "idxgh"
  (delta)/2 -> Bus Creator/10  "fd"
  (delta)/1 -> Bus Creator/9  "idxd"
  Gain2/1 -> (ground height)/1
  Gain/1 -> (altitude)/1
  p,q,r [ras/s]/1 -> Dynamic Contribution/5(omega [rad/s])
  Length Conversion2/1 -> Gain2/1
  Length Conversion1/1 -> Gain/1
  grnd ht/1 -> Length Conversion2/1
  delta/1 -> Angle Conversion2/1
  h/1 -> Length Conversion1/1
  (Mach)/1 -> Bus Creator/3  "idxm"
  (alpha)/1 -> Bus Creator/1  "idxa"
  Angle Conversion2/1 -> (delta)/1
  V wind/1 -> Aerodynamic Forces and Moments/5
  qbar/1 -> Aerodynamic Forces and Moments/2
  Static Contribution/1(Coef) -> Sum2/1
  Sum2/1 -> Aerodynamic Forces and Moments/1
  Control Contribution/1(Coef) -> Sum2/3
  Bus Creator/1 -> Control Contribution/1(bus), Dynamic Contribution/1(bus), Static Contribution/1(bus)
  alfa [rad]/1 -> Angle Conversion3/1
  Mach/1 -> (Mach)/1
  Aerodynamic Forces and Moments/2 -> Ma/1
  Gain1/1 -> Bus Creator1/2, Control Contribution/2(aileron)  "ail"
  Gain3/1 -> Bus Creator1/1, Control Contribution/3(elevator)  "elv"
  Gain4/1 -> Bus Creator1/3, Control Contribution/4(rudder)  "rdr"
  aileron/1 -> Gain1/1
  elevator/1 -> Gain3/1
  rudder/1 -> Gain4/1
  Bus Creator1/1 -> ctrl [°]/1
  Aerodynamic Forces and Moments/1 -> Fa/1
  Center of Gravity/1 -> Aerodynamic Forces and Moments/3
  Center of Pressure/1 -> Aerodynamic Forces and Moments/4
  Dynamic Contribution/1(Coef) -> Sum2/2
  alfa_dot/1 -> Dynamic Contribution/4(alpha_dot [rad/s])
  alfa1/1 -> Dynamic Contribution/2(alpha [rad])
  TAS [m/s]/1 -> Dynamic Contribution/6(TAS)
  Angle Conversion3/1 -> (alpha)/1
  beta1/1 -> Dynamic Contribution/3(beta [rad])

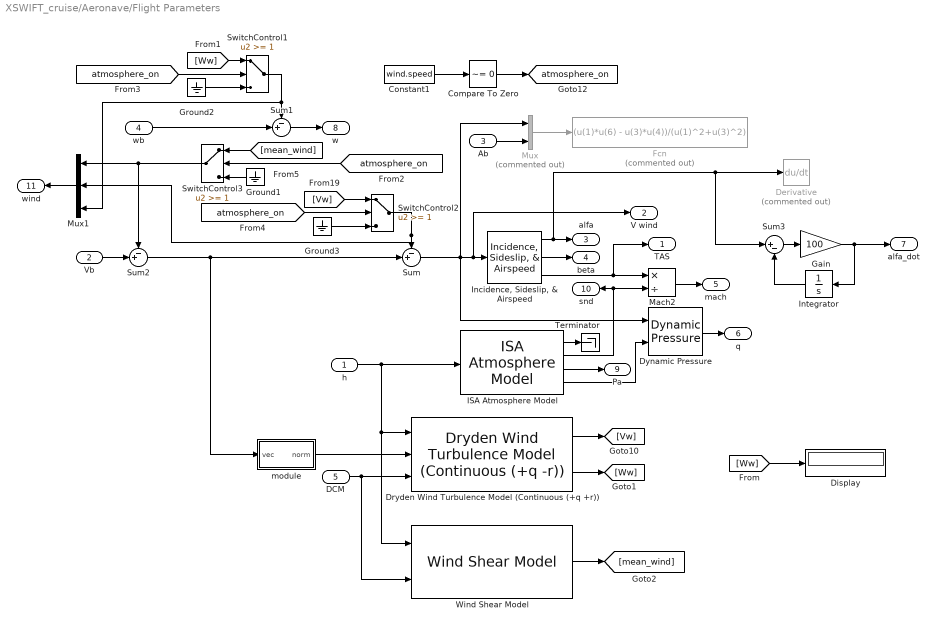
== system XSWIFT_cruise/Aeronave/Flight Parameters ==
  h : Inport
  Vb : Inport  Port=2
  Ab : Inport  Port=3
  wb : Inport  Port=4
  DCM : Inport  Port=5
  Compare To Zero : simulink/Logic and Bit Operations/Compare To Zero  relop=~=  OutDataTypeStr=boolean
  Constant1 : Constant  Value=wind.speed  OutDataTypeStr=boolean
  Derivative : Derivative  Commented=on  CoefficientInTFapproximation=0.01
  Display : Display
  Dryden Wind Turbulence Model (Continuous (+q +r)) : aerolibwind2/Dryden Wind Turbulence Model  (Continuous (+q -r))  units=Metric (MKS)  spec=MIL-F-8785C  model=Continuous Dryden (+q +r)  W20=wind.speed  Wdeg=wind.heading  TurbProb=10^-3 - Moderate  L_high=533.4  Wingspan=data.blref * 12 * 0.0254  ts=0.005  Seed=wind.seeds  T_on=on
  Dynamic Pressure : aerolibasang/Dynamic Pressure
  Fcn : Fcn  Commented=on  Expr=(u(1)*u(6) - u(3)*u(4))/(u(1)^2+u(3)^2)
  Gain : Gain  Gain=100
  Ground1 : Ground
  Ground2 : Ground
  Ground3 : Ground
  ISA Atmosphere Model : aerolibatmos2/ISA Atmosphere Model  useExtended=off  action=None  custom=off  viscosityOut=off  g=9.80665  gamma=1.4  R=287.0531  L=0.0065  h_trop=11000  h_strat=20000  rho0=1.225  P0=101325  T0=288.15  h0=0  S=110.4  Tref=273.15  muref=1.716e-5
  "Incidence, Sideslip, & Airspeed" : aerolibasang/Incidence, Sideslip, & Airspeed
  Integrator : Integrator  InitialCondition=init.alpha
  Mach2 : Product  Inputs=*/  InputSameDT=on  SaturateOnIntegerOverflow=on  OutDataTypeStr=Inherit: Same as first input
  Mux : Mux  Commented=on  Inputs=2
  Mux1 : Mux  Inputs=3
  Sum : Sum  Inputs=-+|
  Sum1 : Sum  Inputs=-+|
  Sum2 : Sum  Inputs=-+|
  Sum3 : Sum  Inputs=|+-
  SwitchControl1 : Switch  Threshold=1  SaturateOnIntegerOverflow=off  InputSameDT=off
  SwitchControl2 : Switch  Threshold=1  SaturateOnIntegerOverflow=off  InputSameDT=off
  SwitchControl3 : Switch  Threshold=1  SaturateOnIntegerOverflow=off  InputSameDT=off
  Terminator : Terminator
  Wind Shear Model : aerolibwind2/Wind Shear Model  units=Metric (MKS)  phase=Category C - Terminal Flight Phase  W_20=wind.speed  Wdeg=wind.heading
  module : Subsystem
  TAS : Outport
  V wind : Outport  Port=2
  alfa : Outport  Port=3
  beta : Outport  Port=4
  mach : Outport  Port=5
  q : Outport  Port=6
  alfa_dot : Outport  Port=7
  w : Outport  Port=8
  Pa : Outport  Port=9
  snd : Outport  Port=10
  wind : Outport  Port=11
  tag scope: atmosphere_on=global
  wires:
  "Incidence, Sideslip, & Airspeed"/3 -> Mach2/1, TAS/1
  ISA Atmosphere Model/1 -> Terminator/1
  ISA Atmosphere Model/3 -> Pa/1
  Mach2/1 -> mach/1
  ISA Atmosphere Model/2 -> snd/1, Mach2/2
  ISA Atmosphere Model/4 -> Dynamic Pressure/2
  "Incidence, Sideslip, & Airspeed"/1 -> Sum3/1, Derivative/1, alfa/1
  "Incidence, Sideslip, & Airspeed"/2 -> beta/1
  Dynamic Pressure/1 -> q/1
  Ab/1 -> Mux/2
  Sum/1 -> Dynamic Pressure/1, V wind/1, "Incidence, Sideslip, & Airspeed"/1, Mux/1
  wb/1 -> Sum1/2
  Sum1/1 -> w/1
  [atmosphere_on] -> SwitchControl1/2
  Ground2/1 -> SwitchControl1/3
  [Ww] -> SwitchControl1/1
  SwitchControl1/1 -> Mux1/3, Sum1/1
  [atmosphere_on] -> SwitchControl2/2
  Ground3/1 -> SwitchControl2/3
  [Vw] -> SwitchControl2/1
  SwitchControl2/1 -> Mux1/2, Sum/1
  Vb/1 -> Sum2/2
  Sum2/1 -> module/1(vec), Sum/2
  SwitchControl3/1 -> Sum2/1, Mux1/1
  [mean_wind] -> SwitchControl3/1
  [atmosphere_on] -> SwitchControl3/2
  Ground1/1 -> SwitchControl3/3
  h/1 -> Wind Shear Model/1, Dryden Wind Turbulence Model (Continuous (+q +r))/1, ISA Atmosphere Model/1
  DCM/1 -> Wind Shear Model/2, Dryden Wind Turbulence Model (Continuous (+q +r))/3
  Dryden Wind Turbulence Model (Continuous (+q +r))/1 -> [Vw]
  Dryden Wind Turbulence Model (Continuous (+q +r))/2 -> [Ww]
  Wind Shear Model/1 -> [mean_wind]
  module/1(norm) -> Dryden Wind Turbulence Model (Continuous (+q +r))/2
  Mux1/1 -> wind/1
  Compare To Zero/1 -> [atmosphere_on]
  Constant1/1 -> Compare To Zero/1
  Mux/1 -> Fcn/1
  Sum3/1 -> Gain/1
  Gain/1 -> alfa_dot/1, Integrator/1
  Integrator/1 -> Sum3/2
  [Ww] -> Display/1

== system XSWIFT_cruise/Aeronave/STOP SIM ==
  sfc : Inport
  vb : Inport  Port=2
  h : Inport  Port=3
  Compare To Constant : simulink/Logic and Bit Operations/Compare To Constant  relop=<=  const=1  OutDataTypeStr=boolean
  Compare To Constant1 : simulink/Logic and Bit Operations/Compare To Constant  relop=>  const=(100*9.81)^2  OutDataTypeStr=boolean
  Compare To Constant2 : simulink/Logic and Bit Operations/Compare To Constant  relop=<  const=0  OutDataTypeStr=boolean
  Display4 : Display
  Dot Product : DotProduct  OutDataTypeStr=Inherit: Inherit via internal rule
  Logical Operator : Logic  Operator=OR  Inputs=3  AllPortsSameDT=off  OutDataTypeStr=boolean
  Mux2 : Mux  Inputs=3
  Selector3 : Selector  InputPortWidth=3  IndexOptions=Index vector (dialog)  Indices=1  OutputSizes=1
  Stop Simulation : Stop
  wires:
  Mux2/1 -> Display4/1
  vb/1 -> Selector3/1
  Compare To Constant2/1 -> Mux2/3, Logical Operator/3
  Compare To Constant1/1 -> Mux2/1, Logical Operator/1
  Selector3/1 -> Compare To Constant/1
  Logical Operator/1 -> Stop Simulation/1
  Compare To Constant/1 -> Mux2/2, Logical Operator/2
  sfc/1 -> Dot Product/1, Dot Product/2
  Dot Product/1 -> Compare To Constant1/1
  h/1 -> Compare To Constant2/1

== system XSWIFT_cruise/Aeronave/actuadores ==
  elev : Inport
  ail : Inport  Port=2
  rdr : Inport  Port=3
  Bus Creator : BusCreator  Inputs=2
  Bus Creator1 : BusCreator  Inputs=2
  Bus Creator2 : BusCreator  Inputs=2
  Scope : Scope  NumInputPorts=3
      settings: ActiveDisplayYMinimum=-0.076306687959086156  ActiveDisplayYMaximum=0.88676019163177566  DataLoggingVariableName=ScopeData5
  ail actuator : aerolibactuator/Nonlinear Second-Order Actuator  wn_fin=data.aler.w  z_fin=0.7  fin_max=1  fin_min=-1  fin_maxrate=inf  fin_act_0=0  fin_act_vel=0
  elev actuator : aerolibactuator/Nonlinear Second-Order Actuator  wn_fin=data.elev.w  z_fin=0.7  fin_max=1  fin_min=-1  fin_maxrate=inf  fin_act_0=init.elv  fin_act_vel=0
  rdr actuator : aerolibactuator/Nonlinear Second-Order Actuator  wn_fin=data.rudr.w  z_fin=0.7  fin_max=1  fin_min=-1  fin_maxrate=inf  fin_act_0=0  fin_act_vel=0
  e_pos : Outport
  a_pos : Outport  Port=2
  r_pos : Outport  Port=3
  wires:
  elev/1 -> Bus Creator/1, elev actuator/1
  ail actuator/1 -> Bus Creator1/2, a_pos/1
  rdr actuator/1 -> Bus Creator2/2, r_pos/1
  rdr/1 -> Bus Creator2/1, rdr actuator/1
  ail/1 -> Bus Creator1/1, ail actuator/1
  elev actuator/1 -> Bus Creator/2, e_pos/1
  Bus Creator/1 -> Scope/1
  Bus Creator1/1 -> Scope/2
  Bus Creator2/1 -> Scope/3

== system XSWIFT_cruise/Aeronave/prop ==
  throtle : Inport
  Constant : Constant  Value=init.thr
  Gain : Gain  Gain=engine.C  Multiplication=Matrix(K*u) (u vector)
  Gain1 : Gain  Gain=engine.A  Multiplication=Matrix(K*u) (u vector)
  Gain2 : Gain  Gain=engine.B  Multiplication=Matrix(K*u) (u vector)
  Integrator : Integrator  InitialConditionSource=external
  Saturation : Saturate  UpperLimit=1  LowerLimit=0
  Scope : Scope  NumInputPorts=2
      settings: ActiveDisplayYMinimum=-0.44270946681321266  ActiveDisplayYMaximum=1.4793642947957946  DataLoggingVariableName=ScopeData4
  Sum : Sum  Inputs=|++
  thrust : Outport
  wires:
  throtle/1 -> Scope/1, Saturation/1  "thr_ref"
  Sum/1 -> Integrator/1
  Gain/1 -> thrust/1  "thrust"
  Integrator/1 -> Scope/2, Gain1/1, Gain/1
  Saturation/1 -> Gain2/1
  Gain2/1 -> Sum/1
  Gain1/1 -> Sum/2
  Constant/1 -> Integrator/2

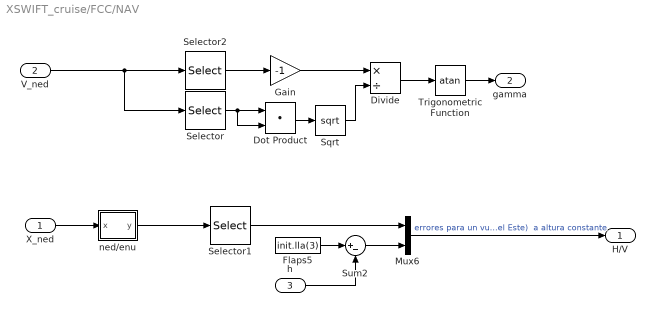
== system XSWIFT_cruise/FCC/NAV ==
  X_ned : Inport
  V_ned : Inport  Port=2
  h : Inport  Port=3
  Divide : Product  Inputs=*/
  Dot Product : DotProduct  OutDataTypeStr=Inherit: Inherit via internal rule
  Flaps5 : Constant  Value=init.lla(3)
  Gain : Gain  Gain=-1
  Mux6 : Mux  Inputs=2
  Selector : Selector  InputPortWidth=3  IndexOptions=Index vector (dialog)  Indices=[1 2]  OutputSizes=1
  Selector1 : Selector  InputPortWidth=3  IndexOptions=Index vector (dialog)  Indices=2  OutputSizes=1
  Selector2 : Selector  InputPortWidth=3  IndexOptions=Index vector (dialog)  Indices=3  OutputSizes=1
  Sqrt : Sqrt
  Sum2 : Sum  Inputs=|+-
  Trigonometric Function : Trigonometry  Operator=atan
  ned/enu : Subsystem
  H/V : Outport
  gamma : Outport  Port=2
  wires:
  Flaps5/1 -> Sum2/1
  Sum2/1 -> Mux6/2
  Mux6/1 -> H/V/1  "errores para un vuelo recto  (hacia el Este)  a altura constante"
  h/1 -> Sum2/2
  X_ned/1 -> ned/enu/1(x)
  Selector1/1 -> Mux6/1
  ned/enu/1(y) -> Selector1/1
  V_ned/1 -> Selector/1, Selector2/1
  Trigonometric Function/1 -> gamma/1
  Selector/1 -> Dot Product/2, Dot Product/1
  Dot Product/1 -> Sqrt/1
  Selector2/1 -> Gain/1
  Sqrt/1 -> Divide/2
  Divide/1 -> Trigonometric Function/1
  Gain/1 -> Divide/1

== system XSWIFT_cruise/FCC/Observador de estados ==
  In1 : Inport
  In2 : Inport  Port=2
  Gain2 : Gain  Gain=- obs_alpha_k'  Multiplication=Matrix(u*K)
  Integrator : Integrator
  Sum2 : Sum  Inputs=-+|
  Sum3 : Sum  Inputs=|++
  l_a : Gain  Gain=obs_alpha_la
  alpha hat : Outport
  wires:
  Integrator/1 -> alpha hat/1, Sum2/1  "alpha hat"
  Sum2/1 -> l_a/1  "error medicion y estimador"
  l_a/1 -> Sum3/1
  In1/1 -> Sum2/2
  Gain2/1 -> Sum3/2  "alpha hat punto"
  Sum3/1 -> Integrator/1  "alpha hat punto"
  In2/1 -> Gain2/1

== system XSWIFT_cruise/FlightGear/phidot, thetadot, psidot ==
  pqr : Inport
  phi theta psi : Inport  Port=2
  Concatenate1 : Concatenate  NumInputs=3
  Concatenate2 : Concatenate  NumInputs=3
  Constant1 : Constant  Commented=on  Value=[0 data.gear.pitch 0]  OutDataTypeStr=single
  SinCos : aerolibobsolete/SinCos
  Sum1 : Sum  Inputs=++|
  phidot : Fcn  Expr=u[1]+(u[2]*u[4]+u[3]*u[7])*(u[5]/u[8])
  psidot : Fcn  Expr=(u[2]*u[4]+u[3]*u[7])/u[8]
  thetadot : Fcn  Expr=u[2]*u[7]-u[3]*u[4]
  ptp_earth : Outport
  ptp_dot : Outport  Port=2
  wires:
  SinCos/2 -> Concatenate1/3
  SinCos/1 -> Concatenate1/2
  Concatenate2/1 -> ptp_dot/1
  phidot/1 -> Concatenate2/1
  thetadot/1 -> Concatenate2/2
  psidot/1 -> Concatenate2/3
  phi theta psi/1 -> Sum1/1, SinCos/1
  pqr/1 -> Concatenate1/1
  Concatenate1/1 -> thetadot/1, phidot/1, psidot/1
  Constant1/1 -> Sum1/2
  Sum1/1 -> ptp_earth/1

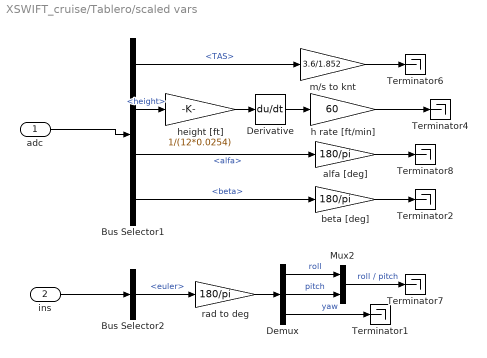
== system XSWIFT_cruise/Tablero/scaled vars ==
  adc : Inport
  ins : Inport  Port=2
  Bus Selector1 : BusSelector  OutputSignals=TAS,height,alfa,beta
  Bus Selector2 : BusSelector  OutputSignals=euler
  Demux : Demux  Outputs=3
  Derivative : Derivative  CoefficientInTFapproximation=0.2
  Mux2 : Mux  Inputs=2
  Terminator{1..2,4,6..8} (6 alike) : Terminator
  alfa [deg] : Gain  Gain=180/pi
  beta [deg] : Gain  Gain=180/pi
  h rate [ft/min] : Gain  Gain=60
  height [ft] : Gain  Gain=1/(12*0.0254)
  m/s to knt : Gain  Gain=3.6/1.852
  rad to deg : Gain  Gain=180/pi
  wires:
  Mux2/1 -> Terminator7/1  "roll / pitch"
  Demux/1 -> Mux2/1  "roll"
  Derivative/1 -> h rate [ft/min]/1
  Bus Selector1/2 -> height [ft]/1  "<height>"
  Demux/3 -> Terminator1/1  "yaw"
  h rate [ft/min]/1 -> Terminator4/1
  adc/1 -> Bus Selector1/1
  ins/1 -> Bus Selector2/1
  Bus Selector1/1 -> m/s to knt/1  "<TAS>"
  height [ft]/1 -> Derivative/1
  Demux/2 -> Mux2/2  "pitch"
  rad to deg/1 -> Demux/1
  alfa [deg]/1 -> Terminator8/1
  m/s to knt/1 -> Terminator6/1
  Bus Selector2/1 -> rad to deg/1  "<euler>"
  Bus Selector1/3 -> alfa [deg]/1  "<alfa>"
  beta [deg]/1 -> Terminator2/1
  Bus Selector1/4 -> beta [deg]/1  "<beta>"

== system XSWIFT_cruise/Aeronave/Aerodinámica/Control Contribution ==
  bus : Inport
  aileron : Inport  Port=2
  elevator : Inport  Port=3
  rudder : Inport  Port=4
  Alerones : Subsystem
  Bus Selector : BusSelector  OutputSignals=idxa,fa
  Elevador : Subsystem
  Mux1 : Mux  Inputs=6
  Rudder : Subsystem
  Sum3 : Sum
  Sum4 : Sum  Inputs=|++
  Coef : Outport
  wires:
  bus/1 -> Bus Selector/1
  Mux1/1 -> Coef/1
  aileron/1 -> Alerones/3(delta)
  Bus Selector/1 -> Elevador/1(idxa), Alerones/1(idxa)  "<idxa>"
  Bus Selector/2 -> Elevador/2(fa), Alerones/2(fa)  "<fa>"
  elevator/1 -> Elevador/3(delta)
  Alerones/2(Cl) -> Mux1/4  "L"
  Elevador/2(CL) -> Mux1/3  "Z"
  Elevador/3(CM) -> Mux1/5  "M"
  Sum3/1 -> Mux1/6  "N"
  Alerones/1(Cn) -> Sum3/1
  rudder/1 -> Rudder/1(delta)
  Rudder/3(Cn) -> Sum3/2
  Elevador/1(CD) -> Sum4/1
  Sum4/1 -> Mux1/1  "X"
  Rudder/1(CD) -> Sum4/2
  Rudder/2(CN) -> Mux1/2  "Y"

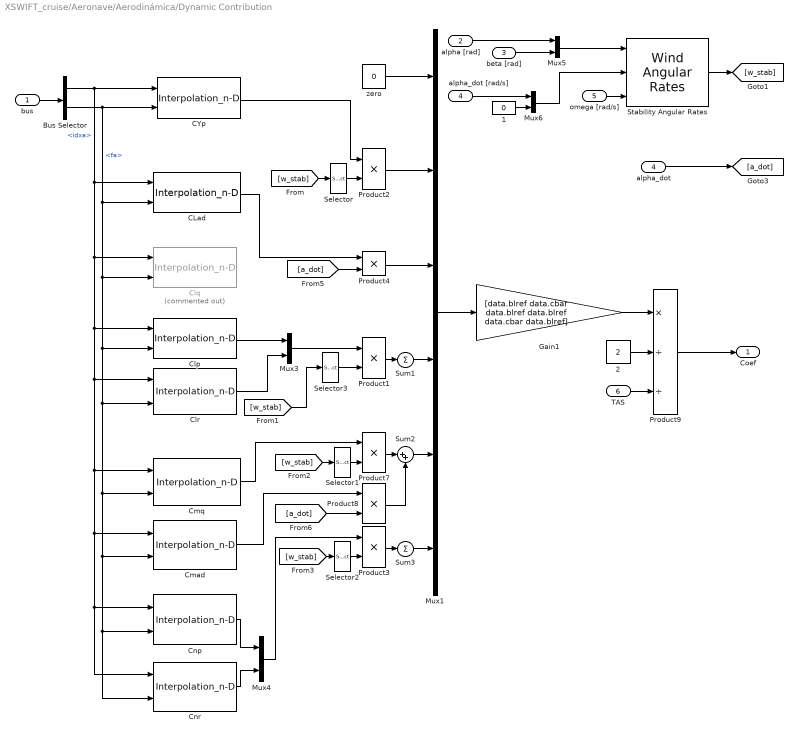
== system XSWIFT_cruise/Aeronave/Aerodinámica/Dynamic Contribution ==
  bus : Inport
  alpha [rad] : Inport  Port=2
  beta [rad] : Inport  Port=3
  alpha_dot [rad/s] : Inport  Port=4
  omega [rad/s] : Inport  Port=5
  TAS : Inport  Port=6
  1 : Constant  Value=0
  2 : Constant  Value=2
  Bus Selector : BusSelector  OutputSignals=idxa,fa
  CLad : Interpolation_n-D  NumberOfTableDimensions=1  Table="permute(data.clad,[1  2])"  OutDataTypeStr=double
      settings: InputPortMap=u0,u1
  CYp : Interpolation_n-D  NumberOfTableDimensions=1  Table="permute(data.cyp,[1  2])"  OutDataTypeStr=double
      settings: InputPortMap=u0,u1
  Clp : Interpolation_n-D  NumberOfTableDimensions=1  Table="permute(data.clp,[1  2])"  OutDataTypeStr=double
      settings: InputPortMap=u0,u1
  Clq : Interpolation_n-D  Commented=on  NumberOfTableDimensions=1  Table="permute(data.clq,[1  2])"  OutDataTypeStr=double
      settings: InputPortMap=u0,u1
  Clr : Interpolation_n-D  NumberOfTableDimensions=1  Table="permute(data.clr,[1  2])"  OutDataTypeStr=double
      settings: InputPortMap=u0,u1
  Cmad : Interpolation_n-D  NumberOfTableDimensions=1  Table="permute(data.cmad,[1  2])"  OutDataTypeStr=double
      settings: InputPortMap=u0,u1
  Cmq : Interpolation_n-D  NumberOfTableDimensions=1  Table="permute(data.cmq,[1  2])"  OutDataTypeStr=double
      settings: InputPortMap=u0,u1
  Cnp : Interpolation_n-D  NumberOfTableDimensions=1  Table="permute(data.cnp,[1  2])"  OutDataTypeStr=double
      settings: InputPortMap=u0,u1
  Cnr : Interpolation_n-D  NumberOfTableDimensions=1  Table="permute(data.cnr,[1  2])"  OutDataTypeStr=double
      settings: InputPortMap=u0,u1
  Gain1 : Gain  Gain=[data.blref data.cbar data.blref data.blref data.cbar data.blref]
  Mux1 : Mux  Inputs=6
  Mux{3..6} (4 alike) : Mux  Inputs=2
  Product{1..4,7..8} (6 alike) : Product  RndMeth=Zero
  Product9 : Product  Inputs=*//  RndMeth=Zero
  Selector : Selector  InputPortWidth=3  IndexOptions=Index vector (dialog)  Indices=1  OutputSizes=1
  Selector1 : Selector  InputPortWidth=3  IndexOptions=Index vector (dialog)  Indices=2  OutputSizes=1
  Selector2 : Selector  InputPortWidth=3  IndexOptions=Index vector (dialog)  Indices=[1 3]  OutputSizes=1
  Selector3 : Selector  InputPortWidth=3  IndexOptions=Index vector (dialog)  Indices=[1 3]  OutputSizes=1
  Stability Angular Rates : aerolibasang/Wind Angular Rates
  Sum1 : Sum  Inputs=+
  Sum2 : Sum  Inputs=|++
  Sum3 : Sum  Inputs=+
  "alpha_dot " : InportShadow  Port=4
  zero : Constant  Value=0
  Coef : Outport
  wires:
  Mux1/1 -> Gain1/1
  CLad/1 -> Product4/1
  Cnp/1 -> Mux4/1
  Cmq/1 -> Product7/1
  Product2/1 -> Mux1/2
  Selector/1 -> Product2/2
  CYp/1 -> Product2/1
  [w_stab] -> Selector/1
  Mux3/1 -> Product1/1
  [w_stab] -> Selector3/1
  Product1/1 -> Sum1/1
  [w_stab] -> Selector1/1
  Selector1/1 -> Product7/2
  Product7/1 -> Sum2/1
  Cmad/1 -> Product8/1
  Product8/1 -> Sum2/2
  [a_dot] -> Product8/2
  Cnr/1 -> Mux4/2
  [w_stab] -> Selector2/1
  Mux4/1 -> Product3/1
  Selector2/1 -> Product3/2
  Sum3/1 -> Mux1/6
  Product3/1 -> Sum3/1
  Gain1/1 -> Product9/1
  Product9/1 -> Coef/1
  2/1 -> Product9/2
  omega [rad/s]/1 -> Stability Angular Rates/3
  Sum2/1 -> Mux1/5
  Product4/1 -> Mux1/3
  zero/1 -> Mux1/1
  alpha [rad]/1 -> Mux5/1
  Mux5/1 -> Stability Angular Rates/1
  Mux6/1 -> Stability Angular Rates/2
  alpha_dot [rad/s]/1 -> Mux6/1
  1/1 -> Mux6/2
  Bus Selector/1 -> CYp/1, CLad/1, Cnr/1, Cnp/1, Cmad/1, Cmq/1, Clr/1, Clp/1, Clq/1  "<idxa>"
  Bus Selector/2 -> CYp/2, CLad/2, Cnr/2, Cnp/2, Cmad/2, Cmq/2, Clr/2, Clp/2, Clq/2  "<fa>"
  bus/1 -> Bus Selector/1
  Clp/1 -> Mux3/1
  Clr/1 -> Mux3/2
  [a_dot] -> Product4/2
  Sum1/1 -> Mux1/4
  TAS/1 -> Product9/3
  "alpha_dot "/1 -> [a_dot]
  Stability Angular Rates/1 -> [w_stab]
  Selector3/1 -> Product1/2
  beta [rad]/1 -> Mux5/2
